simulink model "CLICK_RIO_Simul"  (R2024b)
settings: Solver=VariableStepAuto  StartTime=0.0  StopTime=inf  RelTol=1e-3
libraries: simulink x12, vrlib x7, CLICK_Lib x1
settings Model: Creator=pepev  LastModifiedBy=pepev

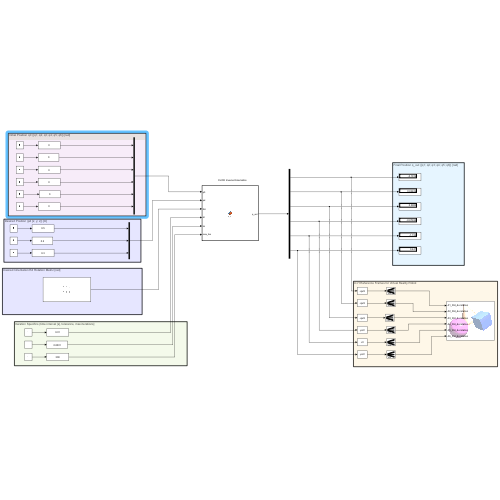
[thumbnail: Simulink's stored preview of the top-level diagram]
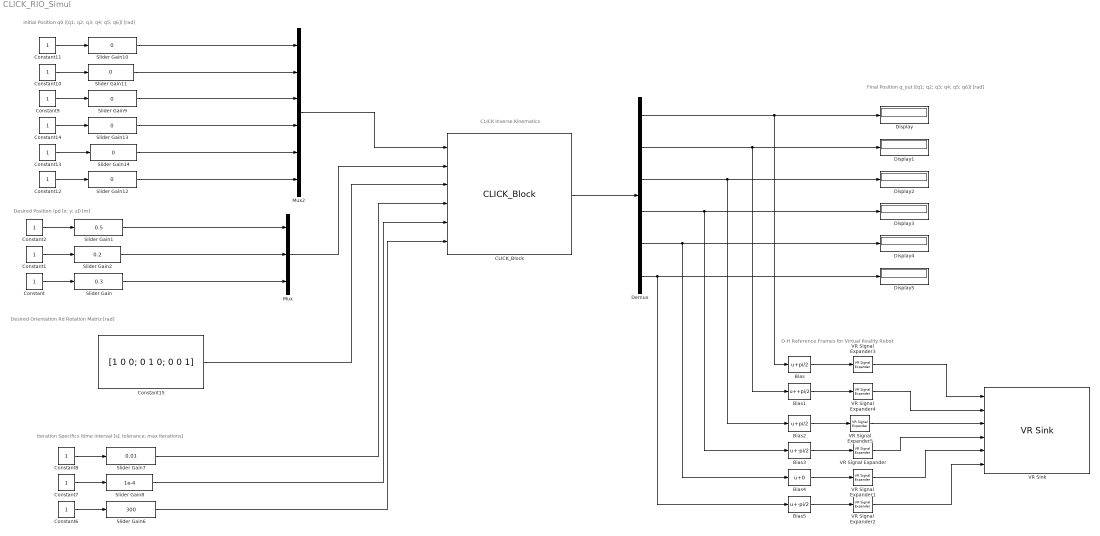
== system CLICK_RIO_Simul ==
  note: CLICK Inverse Kinematics
  note: D-H Reference Frames for Virtual Reality Robot
  note: Final Position q_out ([q1; q2; q3; q4; q5; q6]) [rad]
  note: Iteration Specifics (time interval [s], tolerance, max iterations]
  note: Desired Orientation Rd Rotation Matriz [rad]
  note: Desired Position (pd [x; y; z]) [m]
  note: Initial Position q0 ([q1; q2; q3; q4; q5; q6]) [rad]
  Bias : Bias  Bias=pi/2  SaturateOnIntegerOverflow=off
  Bias1 : Bias  Bias=+pi/2  SaturateOnIntegerOverflow=off
  Bias2 : Bias  Bias=pi/2  SaturateOnIntegerOverflow=off
  Bias3 : Bias  Bias=-pi/2  SaturateOnIntegerOverflow=off
  Bias4 : Bias  SaturateOnIntegerOverflow=off
  Bias5 : Bias  Bias=-pi/2  SaturateOnIntegerOverflow=off
  CLICK_Block : CLICK_Lib/CLICK_Block  SystemSampleTime=-1  VariantActivationTime=update diagram  AllowFlexibleInterface=on  Latency=0  AutoFrameSizeCalculation=off
  Constant{,1..2,6..14} (12 alike) : Constant
  Constant15 : Constant  Value=[1 0 0; 0 1 0; 0 0 1]
  Demux : Demux  Outputs=6
  Display{,1..5} (6 alike) : Display
  Mux : Mux  Inputs=3
  Mux2 : Mux  Inputs=6
  Slider Gain : simulink/Math Operations/Slider Gain  gain=0.3  low=-1  high=1
  Slider Gain1 : simulink/Math Operations/Slider Gain  gain=0.5  low=-3.14  high=3.14
  Slider Gain{10..14} (5 alike) : simulink/Math Operations/Slider Gain  gain=0  low=-3.14  high=3.14
  Slider Gain2 : simulink/Math Operations/Slider Gain  gain=0.2  low=-3.14  high=3.14
  Slider Gain6 : simulink/Math Operations/Slider Gain  gain=300  low=0  high=1000
  Slider Gain7 : simulink/Math Operations/Slider Gain  gain=0.01  low=0  high=3.14
  Slider Gain8 : simulink/Math Operations/Slider Gain  gain=1e-4  low=-3.14  high=3.14
  Slider Gain9 : simulink/Math Operations/Slider Gain  gain=0  low=-1  high=1
  VR Signal Expander{,1..5} (6 alike) : vrlib/VR Signal Expander  outwidth=4  outidx=[4]
  VR Sink : vrlib/VR Sink  InstantiateOnLoad=on  SampleTime=-1  ViewEnable=on  RemoteChange=off  RemoteView=off  FieldsWritten=Jt1_DH_dv.rotation.4.1.1.double#Jt2_DH_dv.rotation.4.1.1.double#Jt3_DH_dv.rotation.4.1.1.double#Jt4_DH_dv.rotation.4.1.1.double#Jt5_DH_dv.rotation.4.1.1.double#Jt6_DH_dv.rotation.4.1.1.double  WorldFileName=vrrobot.wrl  WorldDescription=D-H Reference Frames for Virtual Reality Robot  AutoView=on  VideoDimensions=[]  AllowVariableSize=off
  wires:
  Constant/1 -> Slider Gain/1
  Slider Gain2/1 -> Mux/2
  Constant2/1 -> Slider Gain1/1
  Constant1/1 -> Slider Gain2/1
  Slider Gain1/1 -> Mux/1
  Slider Gain/1 -> Mux/3
  Mux/1 -> CLICK_Block/2
  Constant15/1 -> CLICK_Block/3
  Demux/5 -> Display4/1, Bias4/1
  Bias2/1 -> VR Signal Expander5/1
  VR Signal Expander5/1 -> VR Sink/3
  Bias4/1 -> VR Signal Expander1/1
  VR Signal Expander3/1 -> VR Sink/1
  VR Signal Expander/1 -> VR Sink/4
  Bias3/1 -> VR Signal Expander/1
  Demux/1 -> Bias/1, Display/1
  VR Signal Expander2/1 -> VR Sink/6
  Bias/1 -> VR Signal Expander3/1
  Bias1/1 -> VR Signal Expander4/1
  Demux/2 -> Bias1/1, Display1/1
  VR Signal Expander1/1 -> VR Sink/5
  Bias5/1 -> VR Signal Expander2/1
  Demux/6 -> Bias5/1, Display5/1
  VR Signal Expander4/1 -> VR Sink/2
  Demux/3 -> Bias2/1, Display2/1
  Demux/4 -> Bias3/1, Display3/1
  CLICK_Block/1 -> Demux/1
  Constant7/1 -> Slider Gain8/1
  Constant6/1 -> Slider Gain6/1
  Constant8/1 -> Slider Gain7/1
  Slider Gain7/1 -> CLICK_Block/4
  Slider Gain8/1 -> CLICK_Block/5
  Slider Gain6/1 -> CLICK_Block/6
  Slider Gain12/1 -> Mux2/6
  Slider Gain13/1 -> Mux2/4
  Slider Gain11/1 -> Mux2/2
  Slider Gain14/1 -> Mux2/5
  Slider Gain10/1 -> Mux2/1
  Constant10/1 -> Slider Gain11/1
  Slider Gain9/1 -> Mux2/3
  Constant9/1 -> Slider Gain9/1
  Constant11/1 -> Slider Gain10/1
  Constant12/1 -> Slider Gain12/1
  Constant14/1 -> Slider Gain13/1
  Constant13/1 -> Slider Gain14/1
  Mux2/1 -> CLICK_Block/1
